simulink model "SF021A_HwAgTrajGenn"  (R2013b)
settings: Solver=FixedStepDiscrete  SolverMode=SingleTasking  StartTime=0.0  StopTime=1  FixedStep=0.002  RelTol=1e-3
undefined symbols (not defined in the file): ARCHGLBPRM_2MILLISEC_SEC_F32, HwAgTrajCmdSt1, HwAgTrajGennAgMax, HwAgTrajGennAMax, HwAgTrajGennVelMax, MINATAR_HWDEGPERSECPERSEC_F32, MINVELTAR_HWDEGPERSEC_F32, SYSGLBPRM_HWAGHILIM_HWDEG_F32, SYSGLBPRM_HWAGLOLIM_HWDEG_F32
libraries: simulink x13, NexteerUtilities x5
(part 1 of 2)
settings Model: Creator=DZVCQL  LastModifiedBy=XZB1DB
settings SolverCC: AutoInsertRateTranBlk=on  InsertRTBMode=Always
settings DataIOCC: LimitDataPoints=off  SaveFormat=Structure  ReturnWorkspaceOutputs=on
settings OptimizationCC: BlockReduction=off  InlineParams=on  ZeroExternalMemoryAtStartup=off  ZeroInternalMemoryAtStartup=off  OptimizeModelRefInitCode=on  LifeSpan=1
settings DebuggingCC: SignalInfNanChecking=error  SignalRangeChecking=warning  ReadBeforeWriteMsg=DisableAll  WriteAfterWriteMsg=DisableAll  WriteAfterReadMsg=DisableAll  UnderspecifiedInitializationDetection=Simplified  SolverPrmCheckMsg=error  InheritedTsInSrcMsg=error  DiscreteInheritContinuousMsg=error  SingleTaskRateTransMsg=error  TasksWithSamePriorityMsg=error  SigSpecEnsureSampleTimeMsg=error  CheckMatrixSingularityMsg=error  ParameterUnderflowMsg=error  ParameterPrecisionLossMsg=error  ParameterTunabilityLossMsg=error  FixptConstUnderflowMsg=warning  FixptConstOverflowMsg=warning  VectorMatrixConversionMsg=error  SignalLabelMismatchMsg=error  UnconnectedInputMsg=error  UnconnectedOutputMsg=error  UnconnectedLineMsg=error  SFcnCompatibilityMsg=error  UniqueDataStoreMsg=warning  BusObjectLabelMismatch=error  RootOutportRequireBusObject=error  AssertControl=DisableAll  ModelReferenceIOMsg=error  ModelReferenceVersionMismatchMessage=warning  ModelReferenceIOMismatchMessage=error  ModelReferenceCSMismatchMessage=warning  ModelReferenceDataLoggingMessage=error  StateNameClashWarn=warning  StrictBusMsg=ErrorOnBusTreatedAsVector  NonBusSignalsTreatedAsBus=error  SFUnexpectedBacktrackingDiag=error  SFInvalidInputDataAccessInChartInitDiag=error  SFNoUnconditionalDefaultTransitionDiag=error  SFTransitionOutsideNaturalParentDiag=error  SFUnconditionalTransitionShadowingDiag=error  SFUndirectedBroadcastEventsDiag=error
settings ModelReferenceCC: ModelReferenceNumInstancesAllowed=Single
settings RTWCC: SystemTargetFile=autosar.tlc  GenCodeOnly=on  TemplateMakefile=ert_default_tmf  Description=AUTOSAR  GenerateReport=on  ProcessScript=autosar_make_rtw_hook  LaunchReport=on
settings CodeAppCC: GenerateComments=off  IgnoreCustomStorageClasses=off  CustomSymbolStrType=$N$R$M  CustomSymbolStrBlkIO=$N$M  SimulinkBlockComments=off
settings STFCustomTargetCC: ParMdlRefBuildCompliant=on  CompOptLevelCompliant=on  IncludeMdlTerminateFcn=off  CombineOutputUpdateFcns=on  SuppressErrorStatus=on  ERTFirstTimeCompliant=on  ERTCustomFileBanners=on  SupportNonFinite=off  SupportComplex=off  SupportContinuousTime=off  SupportNonInlinedSFcns=off  MATLABClassNameForMDSCustomization=Simulink.SoftwareTarget.ERTCustomization  AutosarCompliant=on  GRTInterface=off  SystemTargetFile=autosar.tlc
settings ERTTargetCC: CodeReplacementLibrary=ANSI_C  ConcurrentExecutionCompliant=off  IncludeMdlTerminateFcn=off  SuppressErrorStatus=on  SupportNonFinite=off  SupportComplex=off  ModelStepFunctionPrototypeControlCompliant=off  CPPClassGenCompliant=off  AutosarCompliant=on  InlinedParameterPlacement=NonHierarchical  ERTCustomFileTemplate=example_file_process.tlc  EnableUserReplacementTypes=on

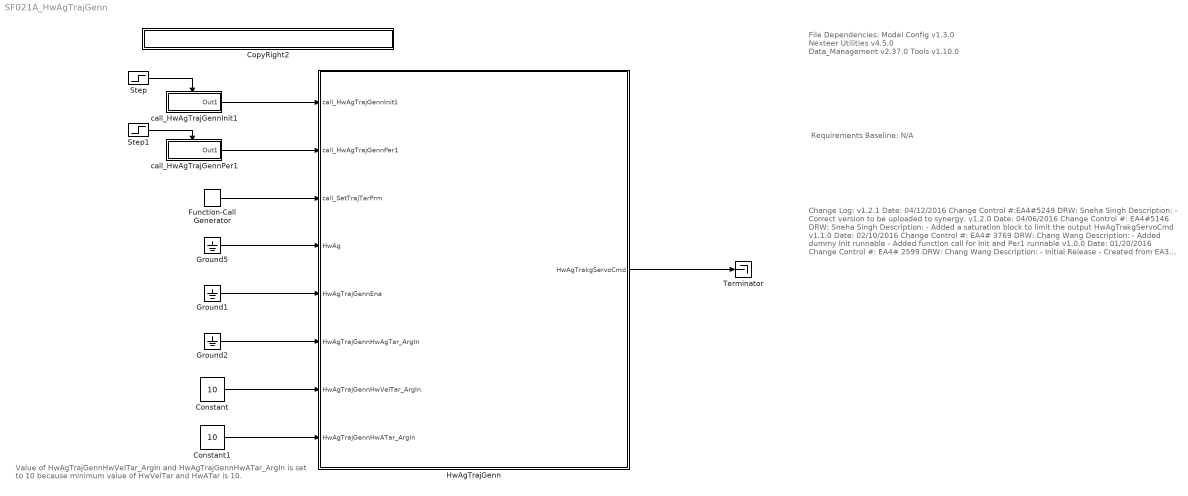
== system SF021A_HwAgTrajGenn ==
  note: Value of HwAgTrajGennHwVelTar_ArgIn and HwAgTrajGennHwATar_ArgIn
      |  is set to 10 because minimum value of HwVelTar and HwATar is 10.
  note: File Dependencies:
      |
      | Model Config v1.3.0
      | Nexteer Utilities v4.5.0
      | Data_Management v2.37.0
      | Tools v1.10.0
  note: Requirements Baseline: N/A
  note: Change Log:
      |
      | v1.2.1
      | Date: 04/12/2016
      | Change Control #:EA4#5249
      | DRW: Sneha Singh
      | Description:
      | - Correct version to be uploaded to synergy.
      |
      | v1.2.0
      | Date: 04/06/2016
      | Change Control #: EA4#5146
      | DRW: Sneha Singh
      | Description:
      | - Added a saturation block to limit the output HwAgTrakgServoCmd
      |
      | v1.1.0
      | Date: 02/10/2016
      | Change Control #: EA4# 3769
      | DRW: Chang Wang
      | Description:
      | - Added dummy Init runnable
      | - Added function call for Init and Per1 runnable
      |
      | v1.0.0
      | Date: 01/20/2016
      | Change Control #: EA4# 2599
      | DRW: Chang Wang
      | Description:
      | - Initial Release
      | - Created from EA3 v002
      | - Level 1 model
  Constant : Constant  Value=10  OutDataTypeStr=single
  Constant1 : Constant  Value=10  OutDataTypeStr=single
  CopyRight2 : Subsystem  Description=|  mask(Copyright Information){none=on}
      | Copyright info block.                                               
      |                                                                     
      | Place copyright information at the top of every subsystem in design.
      mask prompts: none "No parameters"
      mask help: Place copyright information at the top of every subsystem in design.
      mask Display:
      | NxtrConf = 'Nexteer Confidential';
      | 
      | sys = bdroot; %handle for the current model ("system")
      | first = get_param(sys,'Created');
      | if(isempty(first))
      |     first = datestr(now,'yyyy');
      | else
      |     first = first(end-3:end);  %year is last four digits
      | end
      | 
      | last = get_param(sys,'LastModifiedDate');
      | if isempty(last)
      |     last = datestr(now,'yyyy');
      | else
      |     last = last(end-3:end);
      | end
      | 
      | if strcmp(first,last)
      |     fprintf('%s -- Copyright %s Nexteer',NxtrConf,first)
      | else
      |     fprintf('%s -- %s%s- %s Nexteer',NxtrConf,char(169),first,last)
      | end
  Function-Call Generator : simulink/Ports & Subsystems/Function-Call Generator  sample_time=0.002  numberOfIterations=1
  Ground1 : Ground
  Ground2 : Ground
  Ground5 : Ground
  HwAgTrajGenn : Subsystem
  Step : Step  Time=.001  Before=1  After=0  SampleTime=0
  Step1 : Step  Time=.001  SampleTime=0
  Terminator : Terminator
  call_HwAgTrajGennInit1 : Subsystem  TreatAsAtomicUnit=on
  call_HwAgTrajGennPer1 : Subsystem  TreatAsAtomicUnit=on
  wires:
  Ground1/1 -> HwAgTrajGenn/5(HwAgTrajGennEna)
  Ground2/1 -> HwAgTrajGenn/6(HwAgTrajGennHwAgTar_ArgIn)
  Constant/1 -> HwAgTrajGenn/7(HwAgTrajGennHwVelTar_ArgIn)
  HwAgTrajGenn/1(HwAgTrakgServoCmd) -> Terminator/1
  Ground5/1 -> HwAgTrajGenn/4(HwAg)
  Constant1/1 -> HwAgTrajGenn/8(HwAgTrajGennHwATar_ArgIn)
  Function-Call Generator/1 -> HwAgTrajGenn/3(call_SetTrajTarPrm)
  call_HwAgTrajGennInit1/1(Out1) -> HwAgTrajGenn/1(call_HwAgTrajGennInit1)
  Step/1 -> call_HwAgTrajGennInit1/Enable
  Step1/1 -> call_HwAgTrajGennPer1/Enable
  call_HwAgTrajGennPer1/1(Out1) -> HwAgTrajGenn/2(call_HwAgTrajGennPer1)

== system SF021A_HwAgTrajGenn/CopyRight2 ==

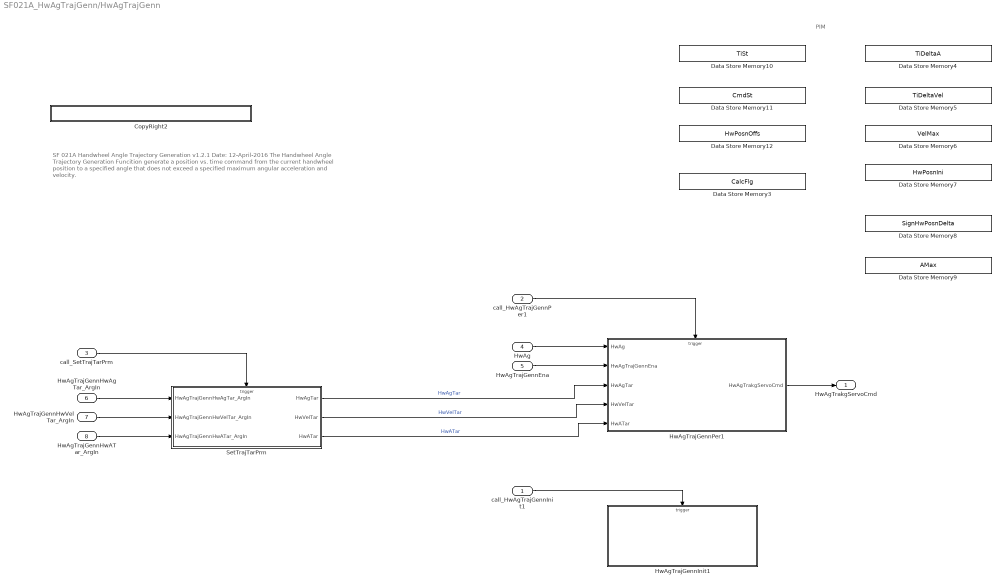
== system SF021A_HwAgTrajGenn/HwAgTrajGenn ==
  note: PIM
  note: SF 021A  Handwheel Angle Trajectory Generation
      | v1.2.1      Date: 12-April-2016
      |
      | The Handwheel Angle Trajectory Generation Funcition generate a position vs. time command from the current handwheel position to a
      | specified angle that does not exceed a specified maximum angular acceleration and velocity.
  call_HwAgTrajGennInit1 : Inport
  call_HwAgTrajGennPer1 : Inport  Port=2
  call_SetTrajTarPrm : Inport  Port=3
  HwAg : Inport  Port=4
  HwAgTrajGennEna : Inport  Port=5
  HwAgTrajGennHwAgTar_ArgIn : Inport  Port=6
  HwAgTrajGennHwVelTar_ArgIn : Inport  Port=7  OutDataTypeStr=single  LockScale=on
  HwAgTrajGennHwATar_ArgIn : Inport  Port=8
  CopyRight2 : Subsystem  Description=|  mask(Copyright Information){none=on}
      | Copyright info block.                                               
      |                                                                     
      | Place copyright information at the top of every subsystem in design.
      mask prompts: none "No parameters"
      mask help: Place copyright information at the top of every subsystem in design.
      mask Display:
      | NxtrConf = 'Nexteer Confidential';
      | 
      | sys = bdroot; %handle for the current model ("system")
      | first = get_param(sys,'Created');
      | if(isempty(first))
      |     first = datestr(now,'yyyy');
      | else
      |     first = first(end-3:end);  %year is last four digits
      | end
      | 
      | last = get_param(sys,'LastModifiedDate');
      | if isempty(last)
      |     last = datestr(now,'yyyy');
      | else
      |     last = last(end-3:end);
      | end
      | 
      | if strcmp(first,last)
      |     fprintf('%s -- Copyright %s Nexteer',NxtrConf,first)
      | else
      |     fprintf('%s -- %s%s- %s Nexteer',NxtrConf,char(169),first,last)
      | end
  Data Store Memory10 : DataStoreMemory  DataStoreName=TiSt  ReadBeforeWriteMsg=warning  WriteAfterWriteMsg=warning  WriteAfterReadMsg=warning  StateMustResolveToSignalObject=on
  Data Store Memory11 : DataStoreMemory  DataStoreName=CmdSt  ReadBeforeWriteMsg=warning  WriteAfterWriteMsg=warning  WriteAfterReadMsg=warning  InitialValue=HwAgTrajCmdSt1.HWAGTRAJCMDST_WAIT  OutDataTypeStr=Enum: HwAgTrajCmdSt1  StateMustResolveToSignalObject=on
  Data Store Memory12 : DataStoreMemory  DataStoreName=HwPosnOffs  ReadBeforeWriteMsg=warning  WriteAfterWriteMsg=warning  WriteAfterReadMsg=warning  StateMustResolveToSignalObject=on
  Data Store Memory3 : DataStoreMemory  DataStoreName=CalcFlg  ReadBeforeWriteMsg=warning  WriteAfterWriteMsg=warning  WriteAfterReadMsg=warning  StateMustResolveToSignalObject=on
  Data Store Memory4 : DataStoreMemory  DataStoreName=TiDeltaA  ReadBeforeWriteMsg=warning  WriteAfterWriteMsg=warning  WriteAfterReadMsg=warning  StateMustResolveToSignalObject=on
  Data Store Memory5 : DataStoreMemory  DataStoreName=TiDeltaVel  ReadBeforeWriteMsg=warning  WriteAfterWriteMsg=warning  WriteAfterReadMsg=warning  StateMustResolveToSignalObject=on
  Data Store Memory6 : DataStoreMemory  DataStoreName=VelMax  ReadBeforeWriteMsg=warning  WriteAfterWriteMsg=warning  WriteAfterReadMsg=warning  StateMustResolveToSignalObject=on
  Data Store Memory7 : DataStoreMemory  DataStoreName=HwPosnIni  ReadBeforeWriteMsg=warning  WriteAfterWriteMsg=warning  WriteAfterReadMsg=warning  StateMustResolveToSignalObject=on
  Data Store Memory8 : DataStoreMemory  DataStoreName=SignHwPosnDelta  ReadBeforeWriteMsg=warning  WriteAfterWriteMsg=warning  WriteAfterReadMsg=warning  StateMustResolveToSignalObject=on
  Data Store Memory9 : DataStoreMemory  DataStoreName=AMax  ReadBeforeWriteMsg=warning  WriteAfterWriteMsg=warning  WriteAfterReadMsg=warning  StateMustResolveToSignalObject=on
  HwAgTrajGennInit1 : Subsystem  TreatAsAtomicUnit=on
  HwAgTrajGennPer1 : Subsystem  TreatAsAtomicUnit=on
  SetTrajTarPrm : Subsystem  TreatAsAtomicUnit=on
  HwAgTrakgServoCmd : Outport
  wires:
  call_SetTrajTarPrm/1 -> SetTrajTarPrm/Trigger
  HwAgTrajGennHwAgTar_ArgIn/1 -> SetTrajTarPrm/1(HwAgTrajGennHwAgTar_ArgIn)
  HwAgTrajGennHwVelTar_ArgIn/1 -> SetTrajTarPrm/2(HwAgTrajGennHwVelTar_ArgIn)
  HwAgTrajGennHwATar_ArgIn/1 -> SetTrajTarPrm/3(HwAgTrajGennHwATar_ArgIn)
  call_HwAgTrajGennPer1/1 -> HwAgTrajGennPer1/Trigger
  HwAg/1 -> HwAgTrajGennPer1/1(HwAg)
  HwAgTrajGennEna/1 -> HwAgTrajGennPer1/2(HwAgTrajGennEna)
  HwAgTrajGennPer1/1(HwAgTrakgServoCmd) -> HwAgTrakgServoCmd/1
  SetTrajTarPrm/1(HwAgTar) -> HwAgTrajGennPer1/3(HwAgTar)  "HwAgTar"
  SetTrajTarPrm/2(HwVelTar) -> HwAgTrajGennPer1/4(HwVelTar)  "HwVelTar"
  SetTrajTarPrm/3(HwATar) -> HwAgTrajGennPer1/5(HwATar)  "HwATar"
  call_HwAgTrajGennInit1/1 -> HwAgTrajGennInit1/Trigger

== system SF021A_HwAgTrajGenn/call_HwAgTrajGennInit1 ==
  Enable : EnablePort
  Function-Call Generator : simulink/Ports & Subsystems/Function-Call Generator  sample_time=.002  numberOfIterations=1
  Out1 : Outport
  wires:
  Function-Call Generator/1 -> Out1/1

== system SF021A_HwAgTrajGenn/call_HwAgTrajGennPer1 ==
  Enable : EnablePort
  call_HwAgTrajGennPer1 : simulink/Ports & Subsystems/Function-Call Generator  RequirementInfo={} %GIDa_c718c7cf_dd39_4fde_b3df_6c879d412d6a  sample_time=0.002  numberOfIterations=1
  Out1 : Outport
  wires:
  call_HwAgTrajGennPer1/1 -> Out1/1

== system SF021A_HwAgTrajGenn/HwAgTrajGenn/CopyRight2 ==

== system SF021A_HwAgTrajGenn/HwAgTrajGenn/HwAgTrajGennInit1 ==
  function : TriggerPort  TriggerType=function-call
  CopyRight2 : Subsystem  Description=|  mask(Copyright Information){none=on}
      | Copyright info block.                                               
      |                                                                     
      | Place copyright information at the top of every subsystem in design.
      mask prompts: none "No parameters"
      mask help: Place copyright information at the top of every subsystem in design.
      mask Display:
      | NxtrConf = 'Nexteer Confidential';
      | 
      | sys = bdroot; %handle for the current model ("system")
      | first = get_param(sys,'Created');
      | if(isempty(first))
      |     first = datestr(now,'yyyy');
      | else
      |     first = first(end-3:end);  %year is last four digits
      | end
      | 
      | last = get_param(sys,'LastModifiedDate');
      | if isempty(last)
      |     last = datestr(now,'yyyy');
      | else
      |     last = last(end-3:end);
      | end
      | 
      | if strcmp(first,last)
      |     fprintf('%s -- Copyright %s Nexteer',NxtrConf,first)
      | else
      |     fprintf('%s -- %s%s- %s Nexteer',NxtrConf,char(169),first,last)
      | end

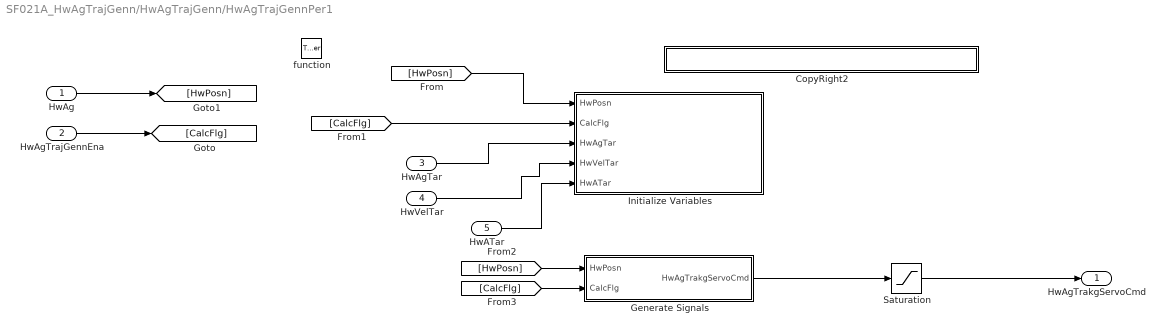
== system SF021A_HwAgTrajGenn/HwAgTrajGenn/HwAgTrajGennPer1 ==
  HwAg : Inport
  HwAgTrajGennEna : Inport  Port=2
  HwAgTar : Inport  Port=3
  HwVelTar : Inport  Port=4
  HwATar : Inport  Port=5
  function : TriggerPort  TriggerType=function-call
  CopyRight2 : Subsystem  Description=|  mask(Copyright Information){none=on}
      | Copyright info block.                                               
      |                                                                     
      | Place copyright information at the top of every subsystem in design.
      mask prompts: none "No parameters"
      mask help: Place copyright information at the top of every subsystem in design.
      mask Display:
      | NxtrConf = 'Nexteer Confidential';
      | 
      | sys = bdroot; %handle for the current model ("system")
      | first = get_param(sys,'Created');
      | if(isempty(first))
      |     first = datestr(now,'yyyy');
      | else
      |     first = first(end-3:end);  %year is last four digits
      | end
      | 
      | last = get_param(sys,'LastModifiedDate');
      | if isempty(last)
      |     last = datestr(now,'yyyy');
      | else
      |     last = last(end-3:end);
      | end
      | 
      | if strcmp(first,last)
      |     fprintf('%s -- Copyright %s Nexteer',NxtrConf,first)
      | else
      |     fprintf('%s -- %s%s- %s Nexteer',NxtrConf,char(169),first,last)
      | end
  Generate Signals : Subsystem
  Initialize Variables : Subsystem  TreatAsAtomicUnit=on
      settings: RTWSystemCode=Nonreusable function
  Saturation : Saturate  UpperLimit=SYSGLBPRM_HWAGHILIM_HWDEG_F32  LowerLimit=SYSGLBPRM_HWAGLOLIM_HWDEG_F32
      settings: AttributesFormatString=|
      | LowerLimit=%<LowerLimit>
      | UpperLimit=%<UpperLimit>
  HwAgTrakgServoCmd : Outport
  wires:
  HwAg/1 -> [HwPosn]
  HwAgTrajGennEna/1 -> [CalcFlg]
  [HwPosn] -> Initialize Variables/1(HwPosn)
  [CalcFlg] -> Initialize Variables/2(CalcFlg)
  [CalcFlg] -> Generate Signals/2(CalcFlg)
  [HwPosn] -> Generate Signals/1(HwPosn)
  Generate Signals/1(HwAgTrakgServoCmd) -> Saturation/1
  HwAgTar/1 -> Initialize Variables/3(HwAgTar)
  HwVelTar/1 -> Initialize Variables/4(HwVelTar)
  HwATar/1 -> Initialize Variables/5(HwATar)
  Saturation/1 -> HwAgTrakgServoCmd/1

== system SF021A_HwAgTrajGenn/HwAgTrajGenn/SetTrajTarPrm ==
  HwAgTrajGennHwAgTar_ArgIn : Inport
  HwAgTrajGennHwVelTar_ArgIn : Inport  Port=2
  HwAgTrajGennHwATar_ArgIn : Inport  Port=3
  function : TriggerPort  TriggerType=function-call
  CopyRight2 : Subsystem  Description=|  mask(Copyright Information){none=on}
      | Copyright info block.                                               
      |                                                                     
      | Place copyright information at the top of every subsystem in design.
      mask prompts: none "No parameters"
      mask help: Place copyright information at the top of every subsystem in design.
      mask Display:
      | NxtrConf = 'Nexteer Confidential';
      | 
      | sys = bdroot; %handle for the current model ("system")
      | first = get_param(sys,'Created');
      | if(isempty(first))
      |     first = datestr(now,'yyyy');
      | else
      |     first = first(end-3:end);  %year is last four digits
      | end
      | 
      | last = get_param(sys,'LastModifiedDate');
      | if isempty(last)
      |     last = datestr(now,'yyyy');
      | else
      |     last = last(end-3:end);
      | end
      | 
      | if strcmp(first,last)
      |     fprintf('%s -- Copyright %s Nexteer',NxtrConf,first)
      | else
      |     fprintf('%s -- %s%s- %s Nexteer',NxtrConf,char(169),first,last)
      | end
  HwAgTar : Outport
  HwVelTar : Outport  Port=2
  HwATar : Outport  Port=3
  wires:
  HwAgTrajGennHwVelTar_ArgIn/1 -> HwVelTar/1
  HwAgTrajGennHwATar_ArgIn/1 -> HwATar/1
  HwAgTrajGennHwAgTar_ArgIn/1 -> HwAgTar/1

== system SF021A_HwAgTrajGenn/HwAgTrajGenn/HwAgTrajGennInit1/CopyRight2 ==

== system SF021A_HwAgTrajGenn/HwAgTrajGenn/HwAgTrajGennPer1/CopyRight2 ==

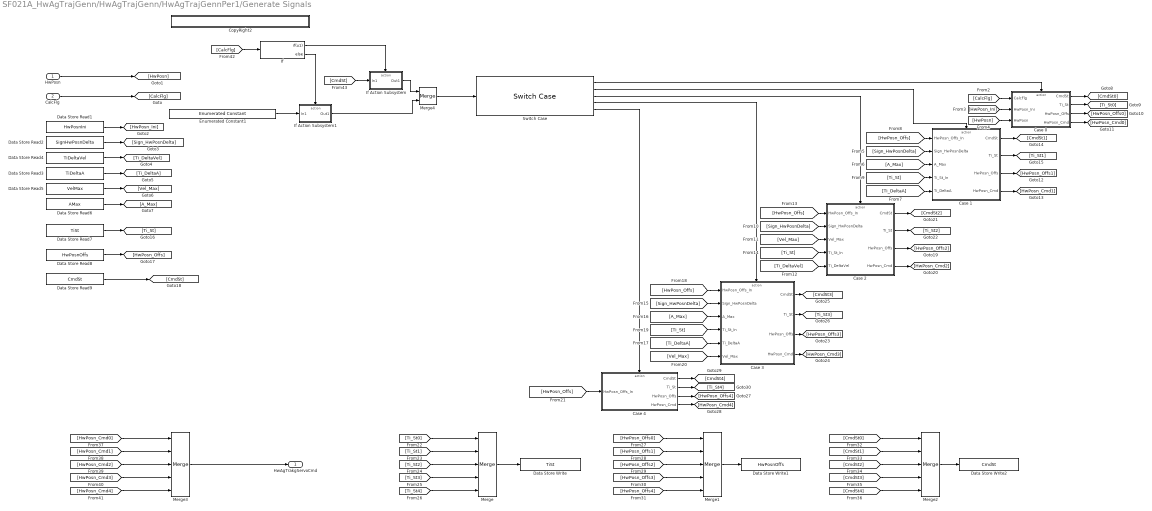
== system SF021A_HwAgTrajGenn/HwAgTrajGenn/HwAgTrajGennPer1/Generate Signals ==
  HwPosn : Inport
  CalcFlg : Inport  Port=2
  Case 0 : Subsystem  TreatAsAtomicUnit=on
  Case 1 : Subsystem  TreatAsAtomicUnit=on
  Case 2 : Subsystem  TreatAsAtomicUnit=on
  Case 3 : Subsystem  TreatAsAtomicUnit=on
  Case 4 : Subsystem  TreatAsAtomicUnit=on
  CopyRight2 : Subsystem  Description=|  mask(Copyright Information){none=on}
      | Copyright info block.                                               
      |                                                                     
      | Place copyright information at the top of every subsystem in design.
      mask prompts: none "No parameters"
      mask help: Place copyright information at the top of every subsystem in design.
      mask Display:
      | NxtrConf = 'Nexteer Confidential';
      | 
      | sys = bdroot; %handle for the current model ("system")
      | first = get_param(sys,'Created');
      | if(isempty(first))
      |     first = datestr(now,'yyyy');
      | else
      |     first = first(end-3:end);  %year is last four digits
      | end
      | 
      | last = get_param(sys,'LastModifiedDate');
      | if isempty(last)
      |     last = datestr(now,'yyyy');
      | else
      |     last = last(end-3:end);
      | end
      | 
      | if strcmp(first,last)
      |     fprintf('%s -- Copyright %s Nexteer',NxtrConf,first)
      | else
      |     fprintf('%s -- %s%s- %s Nexteer',NxtrConf,char(169),first,last)
      | end
  Data Store Read1 : DataStoreRead  DataStoreName=HwPosnIni
  Data Store Read2 : DataStoreRead  DataStoreName=SignHwPosnDelta
  Data Store Read3 : DataStoreRead  DataStoreName=TiDeltaA
  Data Store Read4 : DataStoreRead  DataStoreName=TiDeltaVel
  Data Store Read5 : DataStoreRead  DataStoreName=VelMax
  Data Store Read6 : DataStoreRead  DataStoreName=AMax
  Data Store Read7 : DataStoreRead  Priority=1  DataStoreName=TiSt
      settings: AttributesFormatString="priority:  %<Priority>"
  Data Store Read8 : DataStoreRead  Priority=1  DataStoreName=HwPosnOffs
      settings: AttributesFormatString="priority:  %<Priority>"
  Data Store Read9 : DataStoreRead  Priority=1  DataStoreName=CmdSt
      settings: AttributesFormatString="priority:  %<Priority>"
  Data Store Write : DataStoreWrite  Priority=2  DataStoreName=TiSt
      settings: AttributesFormatString="priority:  %<Priority>"
  Data Store Write1 : DataStoreWrite  Priority=2  DataStoreName=HwPosnOffs
      settings: AttributesFormatString="priority:  %<Priority>"
  Data Store Write2 : DataStoreWrite  Priority=2  DataStoreName=CmdSt
      settings: AttributesFormatString="priority:  %<Priority>"
  Enumerated Constant1 : simulink/Sources/Enumerated Constant  OutDataTypeStr=Enum: HwAgTrajCmdSt1  Value=HwAgTrajCmdSt1.HWAGTRAJCMDST_WAIT  SampleTime=inf
  If : If  IfExpression=u1
  If Action Subsystem : Subsystem  TreatAsAtomicUnit=on
  If Action Subsystem1 : Subsystem  TreatAsAtomicUnit=on
  Merge{,1..3} (4 alike) : Merge  Inputs=5
  Merge4 : Merge
  Switch Case : SwitchCase  CaseConditions={HwAgTrajCmdSt1.HWAGTRAJCMDST_WAIT,HwAgTrajCmdSt1.HWAGTRAJCMDST_HWAGA,HwAgTrajCmdSt1.HWAGTRAJCMDST_CONVEL,HwAgTrajCmdSt1.HWAGTRAJCMDST_HWAGDECEL,HwAgTrajCmdSt1.HWAGTRAJCMDST_HLD}  ShowDefaultCase=off
  HwAgTrakgServoCmd : Outport
  wires:
  CalcFlg/1 -> [CalcFlg]
  HwPosn/1 -> [HwPosn]
  Data Store Read1/1 -> [HwPosn_Ini]
  Data Store Read6/1 -> [A_Max]
  Data Store Read5/1 -> [Vel_Max]
  Data Store Read3/1 -> [Ti_DeltaA]
  Data Store Read4/1 -> [Ti_DeltaVel]
  Data Store Read2/1 -> [Sign_HwPosnDelta]
  Switch Case/1 -> Case 0/Action
  [CalcFlg] -> Case 0/1(CalcFlg)
  [HwPosn_Ini] -> Case 0/2(HwPosn_Ini)
  [HwPosn] -> Case 0/3(HwPosn)
  Case 0/1("CmdSt ") -> [CmdSt0]
  Case 0/2(Ti_St) -> [Ti_St0]
  Case 0/3(HwPosn_Offs) -> [HwPosn_Offs0]
  Case 0/4(HwPosn_Cmd) -> [HwPosn_Cmd0]
  Switch Case/2 -> Case 1/Action
  Case 1/1("CmdSt ") -> [CmdSt1]
  Case 1/2(Ti_St) -> [Ti_St1]
  Case 1/3(HwPosn_Offs) -> [HwPosn_Offs1]
  Case 1/4(HwPosn_Cmd) -> [HwPosn_Cmd1]
  [HwPosn_Offs] -> Case 1/1(HwPosn_Offs_In)
  [A_Max] -> Case 1/3("A_Max ")
  [Sign_HwPosnDelta] -> Case 1/2(Sign_HwPosnDelta)
  [Ti_DeltaA] -> Case 1/5(Ti_DeltaA)
  Data Store Read9/1 -> [CmdSt]
  Data Store Read8/1 -> [HwPosn_Offs]
  Data Store Read7/1 -> [Ti_St]
  [Ti_St] -> Case 1/4(Ti_St_In)
  Case 2/1("CmdSt ") -> [CmdSt2]
  Case 2/2(Ti_St) -> [Ti_St2]
  Case 2/3(HwPosn_Offs) -> [HwPosn_Offs2]
  Case 2/4(HwPosn_Cmd) -> [HwPosn_Cmd2]
  [HwPosn_Offs] -> Case 2/1(HwPosn_Offs_In)
  [Vel_Max] -> Case 2/3("Vel_Max ")
  [Sign_HwPosnDelta] -> Case 2/2(Sign_HwPosnDelta)
  [Ti_DeltaVel] -> Case 2/5(Ti_DeltaVel)
  [Ti_St] -> Case 2/4(Ti_St_In)
  Switch Case/3 -> Case 2/Action
  Case 3/1("CmdSt ") -> [CmdSt3]
  Case 3/2(Ti_St) -> [Ti_St3]
  Case 3/3(HwPosn_Offs) -> [HwPosn_Offs3]
  Case 3/4(HwPosn_Cmd) -> [HwPosn_Cmd3]
  [HwPosn_Offs] -> Case 3/1(HwPosn_Offs_In)
  [A_Max] -> Case 3/3("A_Max ")
  [Sign_HwPosnDelta] -> Case 3/2(Sign_HwPosnDelta)
  [Ti_DeltaA] -> Case 3/5(Ti_DeltaA)
  [Ti_St] -> Case 3/4(Ti_St_In)
  [Vel_Max] -> Case 3/6(Vel_Max)
  Switch Case/4 -> Case 3/Action
  [HwPosn_Offs] -> Case 4/1(HwPosn_Offs_In)
  Case 4/2(Ti_St) -> [Ti_St4]
  Case 4/3(HwPosn_Offs) -> [HwPosn_Offs4]
  Case 4/4(HwPosn_Cmd) -> [HwPosn_Cmd4]
  Case 4/1("CmdSt ") -> [CmdSt4]
  Switch Case/5 -> Case 4/Action
  Merge/1 -> Data Store Write/1
  Merge1/1 -> Data Store Write1/1
  Merge2/1 -> Data Store Write2/1
  [HwPosn_Cmd0] -> Merge3/1
  [HwPosn_Offs0] -> Merge1/1
  [HwPosn_Offs1] -> Merge1/2
  [HwPosn_Offs2] -> Merge1/3
  [HwPosn_Offs3] -> Merge1/4
  [HwPosn_Offs4] -> Merge1/5
  [Ti_St2] -> Merge/3
  [Ti_St4] -> Merge/5
  [Ti_St1] -> Merge/2
  [Ti_St3] -> Merge/4
  [Ti_St0] -> Merge/1
  [HwPosn_Cmd1] -> Merge3/2
  [HwPosn_Cmd2] -> Merge3/3
  [HwPosn_Cmd4] -> Merge3/5
  [HwPosn_Cmd3] -> Merge3/4
  [CmdSt2] -> Merge2/3
  [CmdSt0] -> Merge2/1
  [CmdSt1] -> Merge2/2
  [CmdSt3] -> Merge2/4
  [CmdSt4] -> Merge2/5
  [CalcFlg] -> If/1
  If/1 -> If Action Subsystem/Action
  [CmdSt] -> If Action Subsystem/1(In1)
  Enumerated Constant1/1 -> If Action Subsystem1/1(In1)
  If Action Subsystem/1(Out1) -> Merge4/1
  If Action Subsystem1/1(Out1) -> Merge4/2
  If/2 -> If Action Subsystem1/Action
  Merge4/1 -> Switch Case/1
  Merge3/1 -> HwAgTrakgServoCmd/1

== system SF021A_HwAgTrajGenn/HwAgTrajGenn/HwAgTrajGennPer1/Initialize Variables ==
  HwPosn : Inport
  CalcFlg : Inport  Port=2
  HwAgTar : Inport  Port=3
  HwVelTar : Inport  Port=4
  HwATar : Inport  Port=5
  CopyRight2 : Subsystem  Description=|  mask(Copyright Information){none=on}
      | Copyright info block.                                               
      |                                                                     
      | Place copyright information at the top of every subsystem in design.
      mask prompts: none "No parameters"
      mask help: Place copyright information at the top of every subsystem in design.
      mask Display:
      | NxtrConf = 'Nexteer Confidential';
      | 
      | sys = bdroot; %handle for the current model ("system")
      | first = get_param(sys,'Created');
      | if(isempty(first))
      |     first = datestr(now,'yyyy');
      | else
      |     first = first(end-3:end);  %year is last four digits
      | end
      | 
      | last = get_param(sys,'LastModifiedDate');
      | if isempty(last)
      |     last = datestr(now,'yyyy');
      | else
      |     last = last(end-3:end);
      | end
      | 
      | if strcmp(first,last)
      |     fprintf('%s -- Copyright %s Nexteer',NxtrConf,first)
      | else
      |     fprintf('%s -- %s%s- %s Nexteer',NxtrConf,char(169),first,last)
      | end
  Data Store Read : DataStoreRead  Priority=1  DataStoreName=CalcFlg
      settings: AttributesFormatString="priority:  %<Priority>"
  Data Store Write3 : DataStoreWrite  Priority=2  DataStoreName=CalcFlg
      settings: AttributesFormatString="priority:  %<Priority>"
  If : If  NumInputs=2  IfExpression=~u1 & u2  ShowElse=off
  If Action Subsystem : Subsystem  TreatAsAtomicUnit=on
  wires:
  HwPosn/1 -> If Action Subsystem/1(HwAg)
  If/1 -> If Action Subsystem/Action
  CalcFlg/1 -> Data Store Write3/1, If/2
  Data Store Read/1 -> If/1
  HwAgTar/1 -> If Action Subsystem/2(HwAgTar)
  HwVelTar/1 -> If Action Subsystem/3(HwVelTar)
  HwATar/1 -> If Action Subsystem/4(HwATar)

== system SF021A_HwAgTrajGenn/HwAgTrajGenn/SetTrajTarPrm/CopyRight2 ==

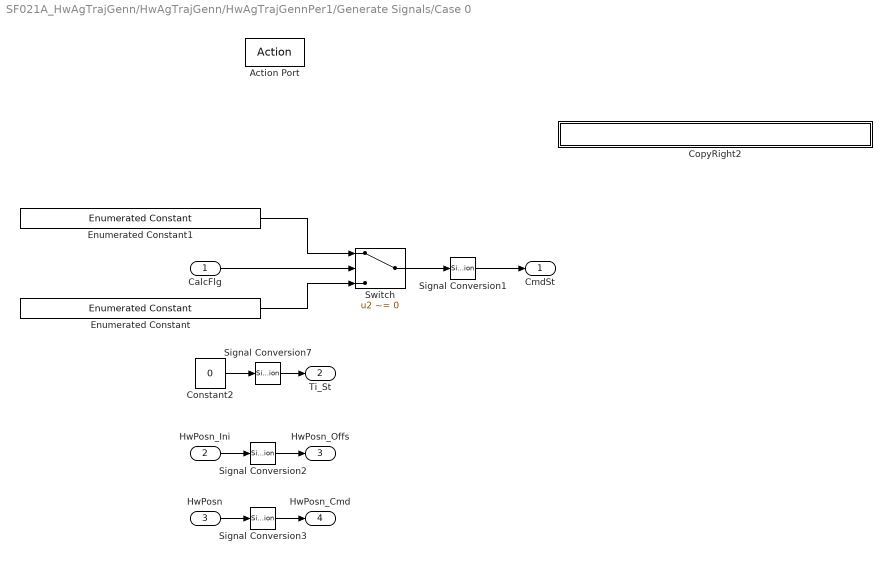
== system SF021A_HwAgTrajGenn/HwAgTrajGenn/HwAgTrajGennPer1/Generate Signals/Case 0 ==
  CalcFlg : Inport
  HwPosn_Ini : Inport  Port=2
  HwPosn : Inport  Port=3
  Action Port : ActionPort  ActionType=case
  Constant2 : Constant  Value=0  OutDataTypeStr=single
  CopyRight2 : Subsystem  Description=|  mask(Copyright Information){none=on}
      | Copyright info block.                                               
      |                                                                     
      | Place copyright information at the top of every subsystem in design.
      mask prompts: none "No parameters"
      mask help: Place copyright information at the top of every subsystem in design.
      mask Display:
      | NxtrConf = 'Nexteer Confidential';
      | 
      | sys = bdroot; %handle for the current model ("system")
      | first = get_param(sys,'Created');
      | if(isempty(first))
      |     first = datestr(now,'yyyy');
      | else
      |     first = first(end-3:end);  %year is last four digits
      | end
      | 
      | last = get_param(sys,'LastModifiedDate');
      | if isempty(last)
      |     last = datestr(now,'yyyy');
      | else
      |     last = last(end-3:end);
      | end
      | 
      | if strcmp(first,last)
      |     fprintf('%s -- Copyright %s Nexteer',NxtrConf,first)
      | else
      |     fprintf('%s -- %s%s- %s Nexteer',NxtrConf,char(169),first,last)
      | end
  Enumerated Constant : simulink/Sources/Enumerated Constant  OutDataTypeStr=Enum: HwAgTrajCmdSt1  Value=HwAgTrajCmdSt1.HWAGTRAJCMDST_WAIT  SampleTime=inf
  Enumerated Constant1 : simulink/Sources/Enumerated Constant  OutDataTypeStr=Enum: HwAgTrajCmdSt1  Value=HwAgTrajCmdSt1.HWAGTRAJCMDST_HWAGA  SampleTime=inf
  Signal Conversion{1..3,7} (4 alike) : SignalConversion
  Switch : Switch  Criteria=u2 ~= 0
  "CmdSt " : Outport
  Ti_St : Outport  Port=2
  HwPosn_Offs : Outport  Port=3
  HwPosn_Cmd : Outport  Port=4
  wires:
  CalcFlg/1 -> Switch/2
  Enumerated Constant1/1 -> Switch/1
  Enumerated Constant/1 -> Switch/3
  Switch/1 -> Signal Conversion1/1
  Constant2/1 -> Signal Conversion7/1
  HwPosn_Ini/1 -> Signal Conversion2/1
  HwPosn/1 -> Signal Conversion3/1
  Signal Conversion7/1 -> Ti_St/1
  Signal Conversion1/1 -> "CmdSt "/1
  Signal Conversion2/1 -> HwPosn_Offs/1
  Signal Conversion3/1 -> HwPosn_Cmd/1

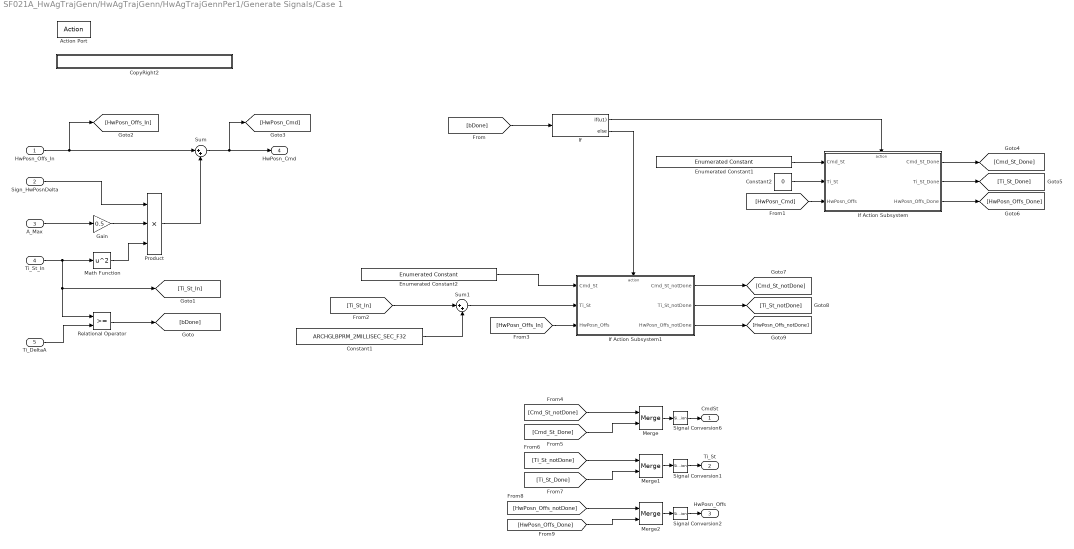
== system SF021A_HwAgTrajGenn/HwAgTrajGenn/HwAgTrajGennPer1/Generate Signals/Case 1 ==
  HwPosn_Offs_In : Inport
  Sign_HwPosnDelta : Inport  Port=2
  "A_Max " : Inport  Port=3
  Ti_St_In : Inport  Port=4
  Ti_DeltaA : Inport  Port=5
  Action Port : ActionPort  ActionType=case
  Constant1 : Constant  Value=ARCHGLBPRM_2MILLISEC_SEC_F32
  Constant2 : Constant  Value=0  OutDataTypeStr=single
  CopyRight2 : Subsystem  Description=|  mask(Copyright Information){none=on}
      | Copyright info block.                                               
      |                                                                     
      | Place copyright information at the top of every subsystem in design.
      mask prompts: none "No parameters"
      mask help: Place copyright information at the top of every subsystem in design.
      mask Display:
      | NxtrConf = 'Nexteer Confidential';
      | 
      | sys = bdroot; %handle for the current model ("system")
      | first = get_param(sys,'Created');
      | if(isempty(first))
      |     first = datestr(now,'yyyy');
      | else
      |     first = first(end-3:end);  %year is last four digits
      | end
      | 
      | last = get_param(sys,'LastModifiedDate');
      | if isempty(last)
      |     last = datestr(now,'yyyy');
      | else
      |     last = last(end-3:end);
      | end
      | 
      | if strcmp(first,last)
      |     fprintf('%s -- Copyright %s Nexteer',NxtrConf,first)
      | else
      |     fprintf('%s -- %s%s- %s Nexteer',NxtrConf,char(169),first,last)
      | end
  Enumerated Constant1 : simulink/Sources/Enumerated Constant  OutDataTypeStr=Enum: HwAgTrajCmdSt1  Value=HwAgTrajCmdSt1.HWAGTRAJCMDST_CONVEL  SampleTime=inf
  Enumerated Constant2 : simulink/Sources/Enumerated Constant  OutDataTypeStr=Enum: HwAgTrajCmdSt1  Value=HwAgTrajCmdSt1.HWAGTRAJCMDST_HWAGA  SampleTime=inf
  Gain : Gain  Gain=0.5
  If : If  IfExpression=u1
  If Action Subsystem : Subsystem  TreatAsAtomicUnit=on
  If Action Subsystem1 : Subsystem  TreatAsAtomicUnit=on
  Math Function : Math  Operator=square  SaturateOnIntegerOverflow=on
  Merge : Merge
  Merge1 : Merge
  Merge2 : Merge
  Product : Product  Inputs=3
  Relational Operator : RelationalOperator  OutDataTypeStr=boolean
  Signal Conversion1 : SignalConversion
  Signal Conversion2 : SignalConversion
  Signal Conversion6 : SignalConversion
  Sum : Sum  Inputs=|++
  Sum1 : Sum  Inputs=|++
  "CmdSt " : Outport
  Ti_St : Outport  Port=2
  HwPosn_Offs : Outport  Port=3
  HwPosn_Cmd : Outport  Port=4
  wires:
  "A_Max "/1 -> Gain/1
  Gain/1 -> Product/2
  Sign_HwPosnDelta/1 -> Product/1
  Ti_St_In/1 -> Relational Operator/1, [Ti_St_In], Math Function/1
  Math Function/1 -> Product/3
  HwPosn_Offs_In/1 -> [HwPosn_Offs_In], Sum/1
  Product/1 -> Sum/2
  Sum/1 -> [HwPosn_Cmd], HwPosn_Cmd/1
  Ti_DeltaA/1 -> Relational Operator/2
  Relational Operator/1 -> [bDone]
  [bDone] -> If/1
  If/1 -> If Action Subsystem/Action
  If/2 -> If Action Subsystem1/Action
  Constant2/1 -> If Action Subsystem/2(Ti_St)
  Enumerated Constant2/1 -> If Action Subsystem1/1(Cmd_St)
  Enumerated Constant1/1 -> If Action Subsystem/1(Cmd_St)
  [HwPosn_Cmd] -> If Action Subsystem/3(HwPosn_Offs)
  [HwPosn_Offs_In] -> If Action Subsystem1/3(HwPosn_Offs)
  If Action Subsystem/1(Cmd_St_Done) -> [Cmd_St_Done]
  If Action Subsystem/2(Ti_St_Done) -> [Ti_St_Done]
  If Action Subsystem/3(HwPosn_Offs_Done) -> [HwPosn_Offs_Done]
  If Action Subsystem1/1(Cmd_St_notDone) -> [Cmd_St_notDone]
  If Action Subsystem1/2(Ti_St_notDone) -> [Ti_St_notDone]
  If Action Subsystem1/3(HwPosn_Offs_notDone) -> [HwPosn_Offs_notDone]
  [Ti_St_In] -> Sum1/1
  Constant1/1 -> Sum1/2
  Sum1/1 -> If Action Subsystem1/2(Ti_St)
  Merge/1 -> Signal Conversion6/1
  Merge1/1 -> Signal Conversion1/1
  Merge2/1 -> Signal Conversion2/1
  [Cmd_St_notDone] -> Merge/1
  [Cmd_St_Done] -> Merge/2
  [Ti_St_notDone] -> Merge1/1
  [Ti_St_Done] -> Merge1/2
  [HwPosn_Offs_notDone] -> Merge2/1
  [HwPosn_Offs_Done] -> Merge2/2
  Signal Conversion6/1 -> "CmdSt "/1
  Signal Conversion1/1 -> Ti_St/1
  Signal Conversion2/1 -> HwPosn_Offs/1

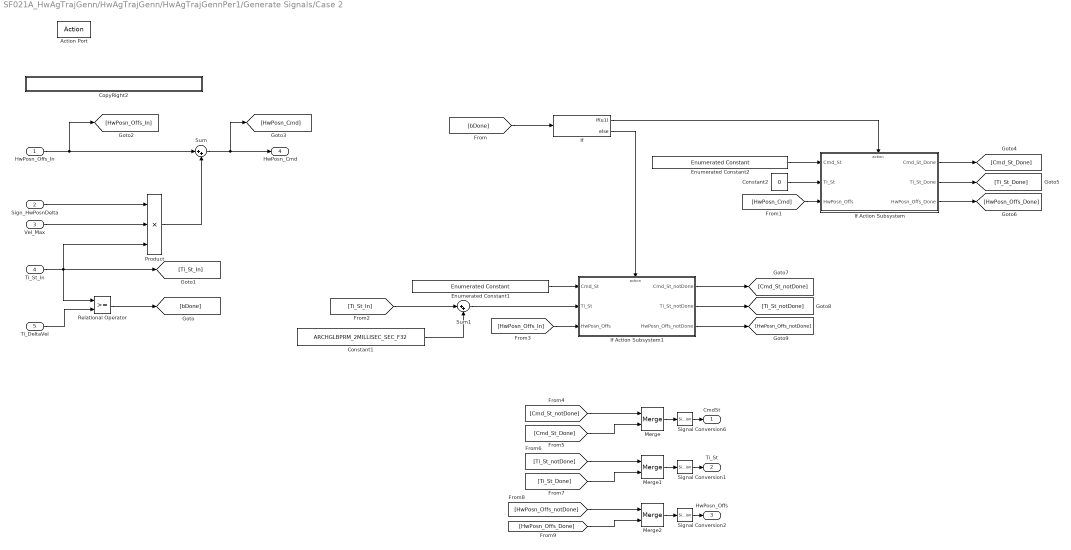
== system SF021A_HwAgTrajGenn/HwAgTrajGenn/HwAgTrajGennPer1/Generate Signals/Case 2 ==
  HwPosn_Offs_In : Inport
  Sign_HwPosnDelta : Inport  Port=2
  "Vel_Max " : Inport  Port=3
  Ti_St_In : Inport  Port=4
  Ti_DeltaVel : Inport  Port=5
  Action Port : ActionPort  ActionType=case
  Constant1 : Constant  Value=ARCHGLBPRM_2MILLISEC_SEC_F32
  Constant2 : Constant  Value=0  OutDataTypeStr=single
  CopyRight2 : Subsystem  Description=|  mask(Copyright Information){none=on}
      | Copyright info block.                                               
      |                                                                     
      | Place copyright information at the top of every subsystem in design.
      mask prompts: none "No parameters"
      mask help: Place copyright information at the top of every subsystem in design.
      mask Display:
      | NxtrConf = 'Nexteer Confidential';
      | 
      | sys = bdroot; %handle for the current model ("system")
      | first = get_param(sys,'Created');
      | if(isempty(first))
      |     first = datestr(now,'yyyy');
      | else
      |     first = first(end-3:end);  %year is last four digits
      | end
      | 
      | last = get_param(sys,'LastModifiedDate');
      | if isempty(last)
      |     last = datestr(now,'yyyy');
      | else
      |     last = last(end-3:end);
      | end
      | 
      | if strcmp(first,last)
      |     fprintf('%s -- Copyright %s Nexteer',NxtrConf,first)
      | else
      |     fprintf('%s -- %s%s- %s Nexteer',NxtrConf,char(169),first,last)
      | end
  Enumerated Constant1 : simulink/Sources/Enumerated Constant  OutDataTypeStr=Enum: HwAgTrajCmdSt1  Value=HwAgTrajCmdSt1.HWAGTRAJCMDST_CONVEL  SampleTime=inf
  Enumerated Constant2 : simulink/Sources/Enumerated Constant  OutDataTypeStr=Enum: HwAgTrajCmdSt1  Value=HwAgTrajCmdSt1.HWAGTRAJCMDST_HWAGDECEL  SampleTime=inf
  If : If  IfExpression=u1
  If Action Subsystem : Subsystem  TreatAsAtomicUnit=on
  If Action Subsystem1 : Subsystem  TreatAsAtomicUnit=on
  Merge : Merge
  Merge1 : Merge
  Merge2 : Merge
  Product : Product  Inputs=3
  Relational Operator : RelationalOperator  OutDataTypeStr=boolean
  Signal Conversion1 : SignalConversion
  Signal Conversion2 : SignalConversion
  Signal Conversion6 : SignalConversion
  Sum : Sum  Inputs=|++
  Sum1 : Sum  Inputs=|++
  "CmdSt " : Outport
  Ti_St : Outport  Port=2
  HwPosn_Offs : Outport  Port=3
  HwPosn_Cmd : Outport  Port=4
  wires:
  [HwPosn_Offs_Done] -> Merge2/2
  [HwPosn_Offs_notDone] -> Merge2/1
  [Ti_St_Done] -> Merge1/2
  [Ti_St_notDone] -> Merge1/1
  [Cmd_St_Done] -> Merge/2
  [Cmd_St_notDone] -> Merge/1
  Merge2/1 -> Signal Conversion2/1
  Merge1/1 -> Signal Conversion1/1
  Merge/1 -> Signal Conversion6/1
  Sum1/1 -> If Action Subsystem1/2(Ti_St)
  Constant1/1 -> Sum1/2
  [Ti_St_In] -> Sum1/1
  If Action Subsystem1/3(HwPosn_Offs_notDone) -> [HwPosn_Offs_notDone]
  If Action Subsystem1/2(Ti_St_notDone) -> [Ti_St_notDone]
  If Action Subsystem1/1(Cmd_St_notDone) -> [Cmd_St_notDone]
  If Action Subsystem/3(HwPosn_Offs_Done) -> [HwPosn_Offs_Done]
  If Action Subsystem/2(Ti_St_Done) -> [Ti_St_Done]
  If Action Subsystem/1(Cmd_St_Done) -> [Cmd_St_Done]
  [HwPosn_Offs_In] -> If Action Subsystem1/3(HwPosn_Offs)
  [HwPosn_Cmd] -> If Action Subsystem/3(HwPosn_Offs)
  Enumerated Constant2/1 -> If Action Subsystem/1(Cmd_St)
  Enumerated Constant1/1 -> If Action Subsystem1/1(Cmd_St)
  Constant2/1 -> If Action Subsystem/2(Ti_St)
  If/2 -> If Action Subsystem1/Action
  If/1 -> If Action Subsystem/Action
  [bDone] -> If/1
  Relational Operator/1 -> [bDone]
  Ti_DeltaVel/1 -> Relational Operator/2
  Sum/1 -> HwPosn_Cmd/1, [HwPosn_Cmd]
  Product/1 -> Sum/2
  HwPosn_Offs_In/1 -> Sum/1, [HwPosn_Offs_In]
  Ti_St_In/1 -> Relational Operator/1, [Ti_St_In], Product/3
  Sign_HwPosnDelta/1 -> Product/1
  "Vel_Max "/1 -> Product/2
  Signal Conversion6/1 -> "CmdSt "/1
  Signal Conversion1/1 -> Ti_St/1
  Signal Conversion2/1 -> HwPosn_Offs/1

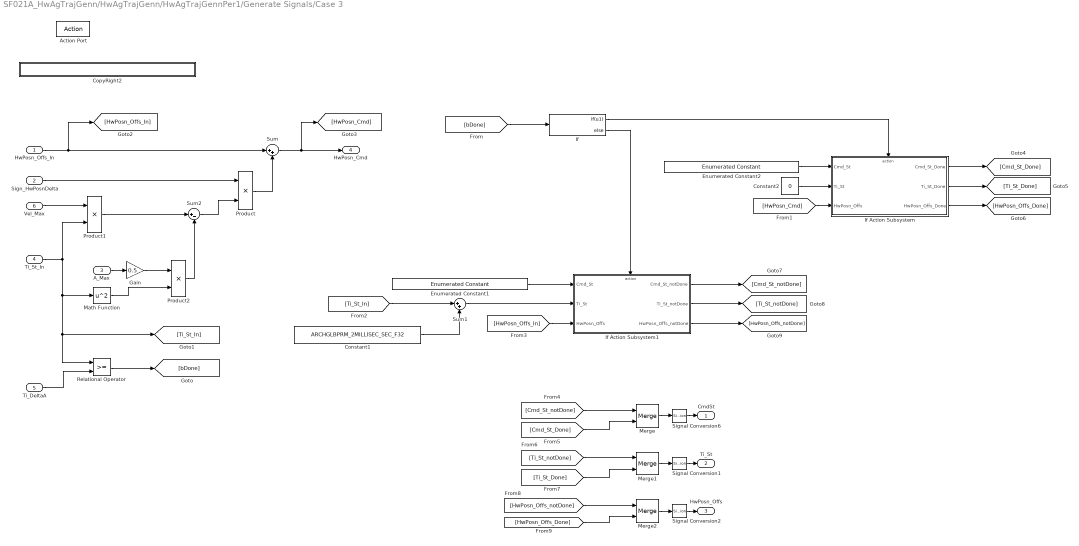
== system SF021A_HwAgTrajGenn/HwAgTrajGenn/HwAgTrajGennPer1/Generate Signals/Case 3 ==
  HwPosn_Offs_In : Inport
  Sign_HwPosnDelta : Inport  Port=2
  "A_Max " : Inport  Port=3
  Ti_St_In : Inport  Port=4
  Ti_DeltaA : Inport  Port=5
  Vel_Max : Inport  Port=6
  Action Port : ActionPort  ActionType=case
  Constant1 : Constant  Value=ARCHGLBPRM_2MILLISEC_SEC_F32
  Constant2 : Constant  Value=0  OutDataTypeStr=single
  CopyRight2 : Subsystem  Description=|  mask(Copyright Information){none=on}
      | Copyright info block.                                               
      |                                                                     
      | Place copyright information at the top of every subsystem in design.
      mask prompts: none "No parameters"
      mask help: Place copyright information at the top of every subsystem in design.
      mask Display:
      | NxtrConf = 'Nexteer Confidential';
      | 
      | sys = bdroot; %handle for the current model ("system")
      | first = get_param(sys,'Created');
      | if(isempty(first))
      |     first = datestr(now,'yyyy');
      | else
      |     first = first(end-3:end);  %year is last four digits
      | end
      | 
      | last = get_param(sys,'LastModifiedDate');
      | if isempty(last)
      |     last = datestr(now,'yyyy');
      | else
      |     last = last(end-3:end);
      | end
      | 
      | if strcmp(first,last)
      |     fprintf('%s -- Copyright %s Nexteer',NxtrConf,first)
      | else
      |     fprintf('%s -- %s%s- %s Nexteer',NxtrConf,char(169),first,last)
      | end
  Enumerated Constant1 : simulink/Sources/Enumerated Constant  OutDataTypeStr=Enum: HwAgTrajCmdSt1  Value=HwAgTrajCmdSt1.HWAGTRAJCMDST_HWAGDECEL  SampleTime=inf
  Enumerated Constant2 : simulink/Sources/Enumerated Constant  OutDataTypeStr=Enum: HwAgTrajCmdSt1  Value=HwAgTrajCmdSt1.HWAGTRAJCMDST_HLD  SampleTime=inf
  Gain : Gain  Gain=0.5
  If : If  IfExpression=u1
  If Action Subsystem : Subsystem  TreatAsAtomicUnit=on
  If Action Subsystem1 : Subsystem  TreatAsAtomicUnit=on
  Math Function : Math  Operator=square  SaturateOnIntegerOverflow=on
  Merge : Merge
  Merge1 : Merge
  Merge2 : Merge
  Product : Product
  Product1 : Product
  Product2 : Product
  Relational Operator : RelationalOperator  OutDataTypeStr=boolean
  Signal Conversion1 : SignalConversion
  Signal Conversion2 : SignalConversion
  Signal Conversion6 : SignalConversion
  Sum : Sum  Inputs=|++
  Sum1 : Sum  Inputs=|++
  Sum2 : Sum  Inputs=|+-
  "CmdSt " : Outport
  Ti_St : Outport  Port=2
  HwPosn_Offs : Outport  Port=3
  HwPosn_Cmd : Outport  Port=4
  wires:
  [HwPosn_Offs_Done] -> Merge2/2
  [HwPosn_Offs_notDone] -> Merge2/1
  [Ti_St_Done] -> Merge1/2
  [Ti_St_notDone] -> Merge1/1
  [Cmd_St_Done] -> Merge/2
  [Cmd_St_notDone] -> Merge/1
  Merge2/1 -> Signal Conversion2/1
  Merge1/1 -> Signal Conversion1/1
  Merge/1 -> Signal Conversion6/1
  Sum1/1 -> If Action Subsystem1/2(Ti_St)
  Constant1/1 -> Sum1/2
  [Ti_St_In] -> Sum1/1
  If Action Subsystem1/3(HwPosn_Offs_notDone) -> [HwPosn_Offs_notDone]
  If Action Subsystem1/2(Ti_St_notDone) -> [Ti_St_notDone]
  If Action Subsystem1/1(Cmd_St_notDone) -> [Cmd_St_notDone]
  If Action Subsystem/3(HwPosn_Offs_Done) -> [HwPosn_Offs_Done]
  If Action Subsystem/2(Ti_St_Done) -> [Ti_St_Done]
  If Action Subsystem/1(Cmd_St_Done) -> [Cmd_St_Done]
  [HwPosn_Offs_In] -> If Action Subsystem1/3(HwPosn_Offs)
  [HwPosn_Cmd] -> If Action Subsystem/3(HwPosn_Offs)
  Enumerated Constant2/1 -> If Action Subsystem/1(Cmd_St)
  Enumerated Constant1/1 -> If Action Subsystem1/1(Cmd_St)
  Constant2/1 -> If Action Subsystem/2(Ti_St)
  If/2 -> If Action Subsystem1/Action
  If/1 -> If Action Subsystem/Action
  [bDone] -> If/1
  Relational Operator/1 -> [bDone]
  Ti_DeltaA/1 -> Relational Operator/2
  Sum/1 -> HwPosn_Cmd/1, [HwPosn_Cmd]
  Product/1 -> Sum/2
  HwPosn_Offs_In/1 -> Sum/1, [HwPosn_Offs_In]
  Math Function/1 -> Product2/2
  Sign_HwPosnDelta/1 -> Product/1
  "A_Max "/1 -> Gain/1
  Vel_Max/1 -> Product1/1
  Ti_St_In/1 -> [Ti_St_In], Relational Operator/1, Math Function/1, Product1/2
  Product1/1 -> Sum2/1
  Gain/1 -> Product2/1
  Product2/1 -> Sum2/2
  Sum2/1 -> Product/2
  Signal Conversion6/1 -> "CmdSt "/1
  Signal Conversion1/1 -> Ti_St/1
  Signal Conversion2/1 -> HwPosn_Offs/1

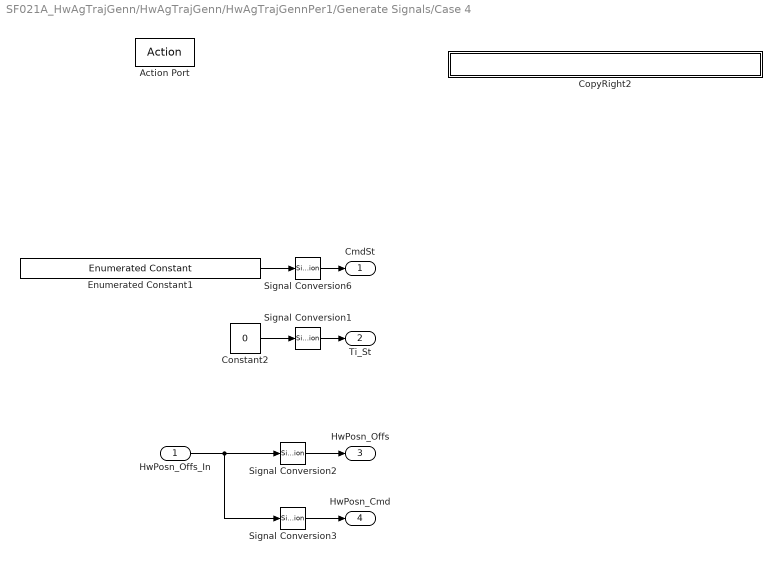
== system SF021A_HwAgTrajGenn/HwAgTrajGenn/HwAgTrajGennPer1/Generate Signals/Case 4 ==
  HwPosn_Offs_In : Inport
  Action Port : ActionPort  ActionType=case
  Constant2 : Constant  Value=0  OutDataTypeStr=single
  CopyRight2 : Subsystem  Description=|  mask(Copyright Information){none=on}
      | Copyright info block.                                               
      |                                                                     
      | Place copyright information at the top of every subsystem in design.
      mask prompts: none "No parameters"
      mask help: Place copyright information at the top of every subsystem in design.
      mask Display:
      | NxtrConf = 'Nexteer Confidential';
      | 
      | sys = bdroot; %handle for the current model ("system")
      | first = get_param(sys,'Created');
      | if(isempty(first))
      |     first = datestr(now,'yyyy');
      | else
      |     first = first(end-3:end);  %year is last four digits
      | end
      | 
      | last = get_param(sys,'LastModifiedDate');
      | if isempty(last)
      |     last = datestr(now,'yyyy');
      | else
      |     last = last(end-3:end);
      | end
      | 
      | if strcmp(first,last)
      |     fprintf('%s -- Copyright %s Nexteer',NxtrConf,first)
      | else
      |     fprintf('%s -- %s%s- %s Nexteer',NxtrConf,char(169),first,last)
      | end
  Enumerated Constant1 : simulink/Sources/Enumerated Constant  OutDataTypeStr=Enum: HwAgTrajCmdSt1  Value=HwAgTrajCmdSt1.HWAGTRAJCMDST_HLD  SampleTime=inf
  Signal Conversion{1..3,6} (4 alike) : SignalConversion
  "CmdSt " : Outport
  Ti_St : Outport  Port=2
  HwPosn_Offs : Outport  Port=3
  HwPosn_Cmd : Outport  Port=4
  wires:
  Constant2/1 -> Signal Conversion1/1
  Enumerated Constant1/1 -> Signal Conversion6/1
  HwPosn_Offs_In/1 -> Signal Conversion3/1, Signal Conversion2/1
  Signal Conversion6/1 -> "CmdSt "/1
  Signal Conversion1/1 -> Ti_St/1
  Signal Conversion2/1 -> HwPosn_Offs/1
  Signal Conversion3/1 -> HwPosn_Cmd/1

== system SF021A_HwAgTrajGenn/HwAgTrajGenn/HwAgTrajGennPer1/Generate Signals/CopyRight2 ==

== system SF021A_HwAgTrajGenn/HwAgTrajGenn/HwAgTrajGennPer1/Generate Signals/If Action Subsystem ==
  In1 : Inport
  Action Port : ActionPort  ActionType=then
  Out1 : Outport
  wires:
  In1/1 -> Out1/1

== system SF021A_HwAgTrajGenn/HwAgTrajGenn/HwAgTrajGennPer1/Generate Signals/If Action Subsystem1 ==
  In1 : Inport
  Action Port : ActionPort  ActionType=else
  Out1 : Outport
  wires:
  In1/1 -> Out1/1

== system SF021A_HwAgTrajGenn/HwAgTrajGenn/HwAgTrajGennPer1/Initialize Variables/CopyRight2 ==

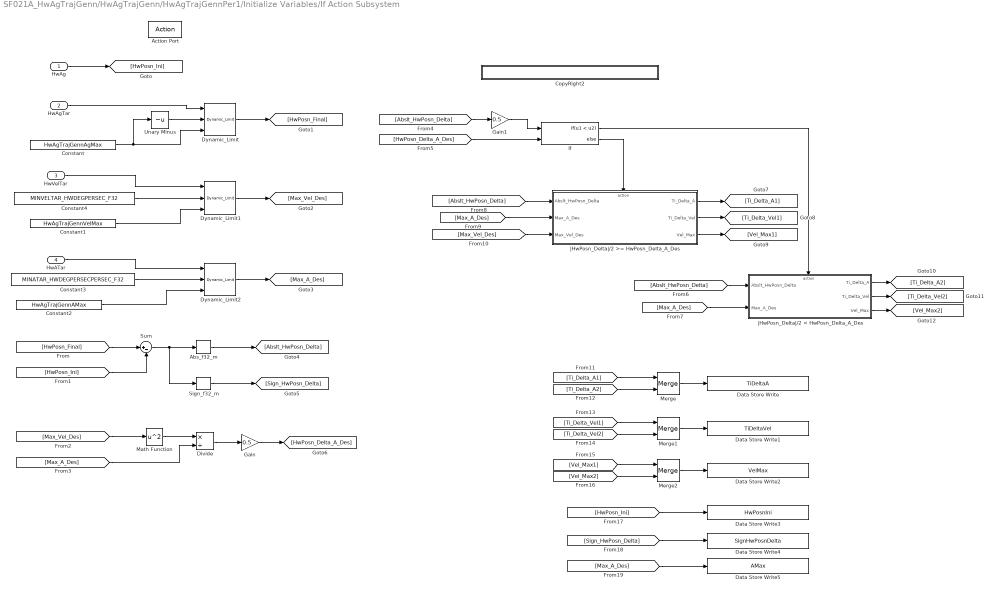
== system SF021A_HwAgTrajGenn/HwAgTrajGenn/HwAgTrajGennPer1/Initialize Variables/If Action Subsystem ==
  HwAg : Inport
  HwAgTar : Inport  Port=2
  HwVelTar : Inport  Port=3
  HwATar : Inport  Port=4
  Action Port : ActionPort  ActionType=then
  Abs_f32_m : NexteerUtilities/Abs_f32_m
      settings: AttributesFormatString=Abs_f32
  Constant : Constant  Value=HwAgTrajGennAgMax
  Constant1 : Constant  Value=HwAgTrajGennVelMax
  Constant2 : Constant  Value=HwAgTrajGennAMax
  Constant3 : Constant  Value=MINATAR_HWDEGPERSECPERSEC_F32
  Constant4 : Constant  Value=MINVELTAR_HWDEGPERSEC_F32
  CopyRight2 : Subsystem  Description=|  mask(Copyright Information){none=on}
      | Copyright info block.                                               
      |                                                                     
      | Place copyright information at the top of every subsystem in design.
      mask prompts: none "No parameters"
      mask help: Place copyright information at the top of every subsystem in design.
      mask Display:
      | NxtrConf = 'Nexteer Confidential';
      | 
      | sys = bdroot; %handle for the current model ("system")
      | first = get_param(sys,'Created');
      | if(isempty(first))
      |     first = datestr(now,'yyyy');
      | else
      |     first = first(end-3:end);  %year is last four digits
      | end
      | 
      | last = get_param(sys,'LastModifiedDate');
      | if isempty(last)
      |     last = datestr(now,'yyyy');
      | else
      |     last = last(end-3:end);
      | end
      | 
      | if strcmp(first,last)
      |     fprintf('%s -- Copyright %s Nexteer',NxtrConf,first)
      | else
      |     fprintf('%s -- %s%s- %s Nexteer',NxtrConf,char(169),first,last)
      | end
  Data Store Write : DataStoreWrite  DataStoreName=TiDeltaA
  Data Store Write1 : DataStoreWrite  DataStoreName=TiDeltaVel
  Data Store Write2 : DataStoreWrite  DataStoreName=VelMax
  Data Store Write3 : DataStoreWrite  DataStoreName=HwPosnIni
  Data Store Write4 : DataStoreWrite  DataStoreName=SignHwPosnDelta
  Data Store Write5 : DataStoreWrite  DataStoreName=AMax
  Divide : Product  Inputs=*/
  Dynamic_Limit : NexteerUtilities/Dynamic_Limit
  Dynamic_Limit1 : NexteerUtilities/Dynamic_Limit
  Dynamic_Limit2 : NexteerUtilities/Dynamic_Limit
  Gain : Gain  Gain=0.5
  Gain1 : Gain  Gain=0.5
  If : If  NumInputs=2  IfExpression=u1 < u2
  Math Function : Math  Operator=square  SaturateOnIntegerOverflow=on
  Merge : Merge
  Merge1 : Merge
  Merge2 : Merge
  Sign_f32_m : NexteerUtilities/Sign_f32_m
      settings: AttributesFormatString=Sign_f32
  Sum : Sum  Inputs=|+-
  Unary Minus : UnaryMinus
  |HwPosn_Delta|/2 < HwPosn_Delta_A_Des : Subsystem  TreatAsAtomicUnit=on
  |HwPosn_Delta|/2 >= HwPosn_Delta_A_Des : Subsystem  TreatAsAtomicUnit=on
  wires:
  HwAg/1 -> [HwPosn_Ini]
  HwAgTar/1 -> Dynamic_Limit/1
  Unary Minus/1 -> Dynamic_Limit/2
  Constant/1 -> Dynamic_Limit/3, Unary Minus/1
  Dynamic_Limit/1 -> [HwPosn_Final]
  HwVelTar/1 -> Dynamic_Limit1/1
  Constant4/1 -> Dynamic_Limit1/2
  Constant1/1 -> Dynamic_Limit1/3
  Dynamic_Limit1/1 -> [Max_Vel_Des]
  HwATar/1 -> Dynamic_Limit2/1
  Constant3/1 -> Dynamic_Limit2/2
  Constant2/1 -> Dynamic_Limit2/3
  Dynamic_Limit2/1 -> [Max_A_Des]
  [HwPosn_Final] -> Sum/1
  [HwPosn_Ini] -> Sum/2
  Sum/1 -> Sign_f32_m/1, Abs_f32_m/1
  Abs_f32_m/1 -> [Abslt_HwPosn_Delta]
  Sign_f32_m/1 -> [Sign_HwPosn_Delta]
  [Max_Vel_Des] -> Math Function/1
  [Max_A_Des] -> Divide/2
  Math Function/1 -> Divide/1
  Divide/1 -> Gain/1
  Gain/1 -> [HwPosn_Delta_A_Des]
  [Abslt_HwPosn_Delta] -> Gain1/1
  [HwPosn_Delta_A_Des] -> If/2
  Gain1/1 -> If/1
  If/1 -> |HwPosn_Delta|/2 < HwPosn_Delta_A_Des/Action
  If/2 -> |HwPosn_Delta|/2 >= HwPosn_Delta_A_Des/Action
  [Abslt_HwPosn_Delta] -> |HwPosn_Delta|/2 < HwPosn_Delta_A_Des/1(Abslt_HwPosn_Delta)
  [Max_A_Des] -> |HwPosn_Delta|/2 < HwPosn_Delta_A_Des/2("Max_A_Des ")
  [Abslt_HwPosn_Delta] -> |HwPosn_Delta|/2 >= HwPosn_Delta_A_Des/1(Abslt_HwPosn_Delta)
  [Max_A_Des] -> |HwPosn_Delta|/2 >= HwPosn_Delta_A_Des/2(Max_A_Des)
  [Max_Vel_Des] -> |HwPosn_Delta|/2 >= HwPosn_Delta_A_Des/3(Max_Vel_Des)
  |HwPosn_Delta|/2 >= HwPosn_Delta_A_Des/1(Ti_Delta_A) -> [Ti_Delta_A1]
  |HwPosn_Delta|/2 >= HwPosn_Delta_A_Des/2(Ti_Delta_Vel) -> [Ti_Delta_Vel1]
  |HwPosn_Delta|/2 >= HwPosn_Delta_A_Des/3(Vel_Max) -> [Vel_Max1]
  |HwPosn_Delta|/2 < HwPosn_Delta_A_Des/1(Ti_Delta_A) -> [Ti_Delta_A2]
  |HwPosn_Delta|/2 < HwPosn_Delta_A_Des/2(Ti_Delta_Vel) -> [Ti_Delta_Vel2]
  |HwPosn_Delta|/2 < HwPosn_Delta_A_Des/3(Vel_Max) -> [Vel_Max2]
  Merge/1 -> Data Store Write/1
  Merge1/1 -> Data Store Write1/1
  Merge2/1 -> Data Store Write2/1
  [HwPosn_Ini] -> Data Store Write3/1
  [Sign_HwPosn_Delta] -> Data Store Write4/1
  [Max_A_Des] -> Data Store Write5/1
  [Ti_Delta_A1] -> Merge/1
  [Ti_Delta_A2] -> Merge/2
  [Ti_Delta_Vel1] -> Merge1/1
  [Ti_Delta_Vel2] -> Merge1/2
  [Vel_Max1] -> Merge2/1
  [Vel_Max2] -> Merge2/2

== system SF021A_HwAgTrajGenn/HwAgTrajGenn/HwAgTrajGennPer1/Generate Signals/Case 0/CopyRight2 ==

== system SF021A_HwAgTrajGenn/HwAgTrajGenn/HwAgTrajGennPer1/Generate Signals/Case 1/CopyRight2 ==

== system SF021A_HwAgTrajGenn/HwAgTrajGenn/HwAgTrajGennPer1/Generate Signals/Case 1/If Action Subsystem ==
  Cmd_St : Inport
  Ti_St : Inport  Port=2
  HwPosn_Offs : Inport  Port=3
  Action Port : ActionPort  ActionType=then
  CopyRight2 : Subsystem  Description=|  mask(Copyright Information){none=on}
      | Copyright info block.                                               
      |                                                                     
      | Place copyright information at the top of every subsystem in design.
      mask prompts: none "No parameters"
      mask help: Place copyright information at the top of every subsystem in design.
      mask Display:
      | NxtrConf = 'Nexteer Confidential';
      | 
      | sys = bdroot; %handle for the current model ("system")
      | first = get_param(sys,'Created');
      | if(isempty(first))
      |     first = datestr(now,'yyyy');
      | else
      |     first = first(end-3:end);  %year is last four digits
      | end
      | 
      | last = get_param(sys,'LastModifiedDate');
      | if isempty(last)
      |     last = datestr(now,'yyyy');
      | else
      |     last = last(end-3:end);
      | end
      | 
      | if strcmp(first,last)
      |     fprintf('%s -- Copyright %s Nexteer',NxtrConf,first)
      | else
      |     fprintf('%s -- %s%s- %s Nexteer',NxtrConf,char(169),first,last)
      | end
  Cmd_St_Done : Outport
  Ti_St_Done : Outport  Port=2
  HwPosn_Offs_Done : Outport  Port=3
  wires:
  Cmd_St/1 -> Cmd_St_Done/1
  Ti_St/1 -> Ti_St_Done/1
  HwPosn_Offs/1 -> HwPosn_Offs_Done/1
